simulink model "gm_model"  (R2022a)
settings: Solver=FixedStepAuto  StartTime=0.0  StopTime=1e2  RelTol=1e-3
settings Model: Creator=mrem  LastModifiedBy=mrem
settings OptimizationCC: BlockReduction=off  ConditionallyExecuteInputs=off
settings DebuggingCC: InheritedTsInSrcMsg=none

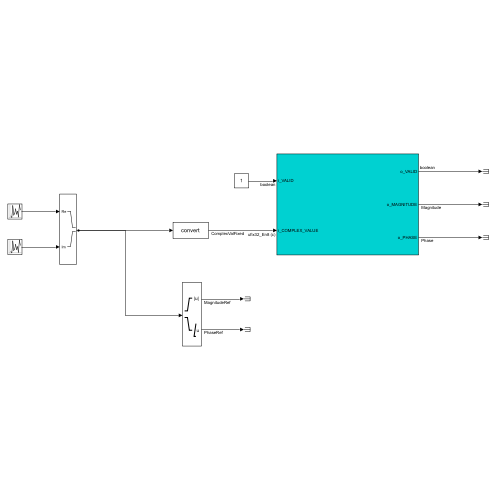
[thumbnail: Simulink's stored preview of the top-level diagram]
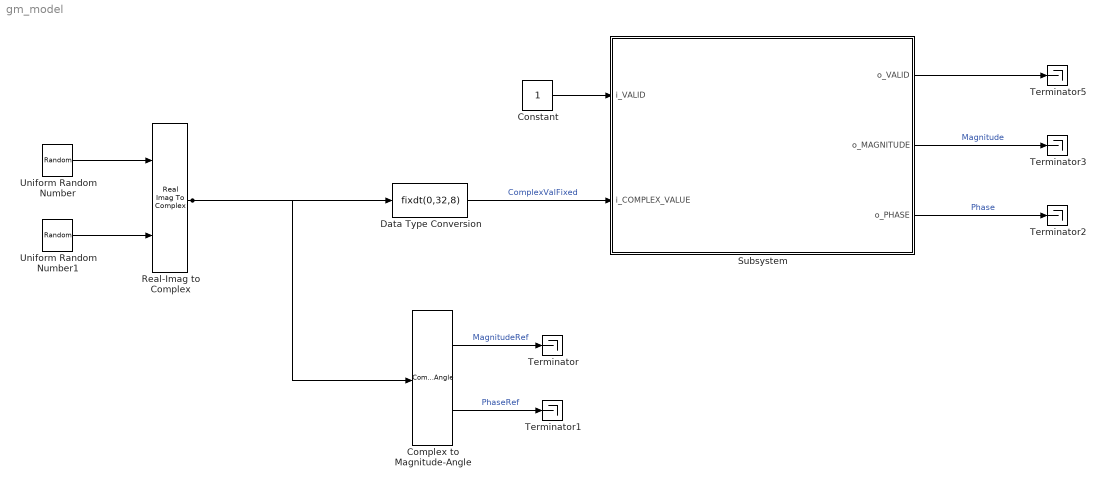
== system gm_model ==
  Complex to Magnitude-Angle : ComplexToMagnitudeAngle
  Constant : Constant  OutDataTypeStr=boolean  SampleTime=-1
  Data Type Conversion : DataTypeConversion  OutDataTypeStr=fixdt(0,32,8)  RndMeth=Round  SaturateOnIntegerOverflow=off
  Real-Imag to Complex : RealImagToComplex
  Subsystem : Subsystem
  Terminator{,1..3,5} (5 alike) : Terminator
  Uniform Random Number : UniformRandomNumber  Minimum=0  Maximum=16777215.9909375  Seed=24  SampleTime=1
  Uniform Random Number1 : UniformRandomNumber  Minimum=0  Maximum=16777215.9909375  Seed=25  SampleTime=1
  wires:
  Data Type Conversion/1 -> Subsystem/2(i_COMPLEX_VALUE)  "ComplexValFixed"
  Subsystem/1(o_VALID) -> Terminator5/1
  Subsystem/3(o_PHASE) -> Terminator2/1  "Phase"
  Subsystem/2(o_MAGNITUDE) -> Terminator3/1  "Magnitude"
  Complex to Magnitude-Angle/2 -> Terminator1/1  "PhaseRef"
  Complex to Magnitude-Angle/1 -> Terminator/1  "MagnitudeRef"
  Real-Imag to Complex/1 -> Data Type Conversion/1, Complex to Magnitude-Angle/1
  Uniform Random Number/1 -> Real-Imag to Complex/1
  Uniform Random Number1/1 -> Real-Imag to Complex/2
  Constant/1 -> Subsystem/1(i_VALID)

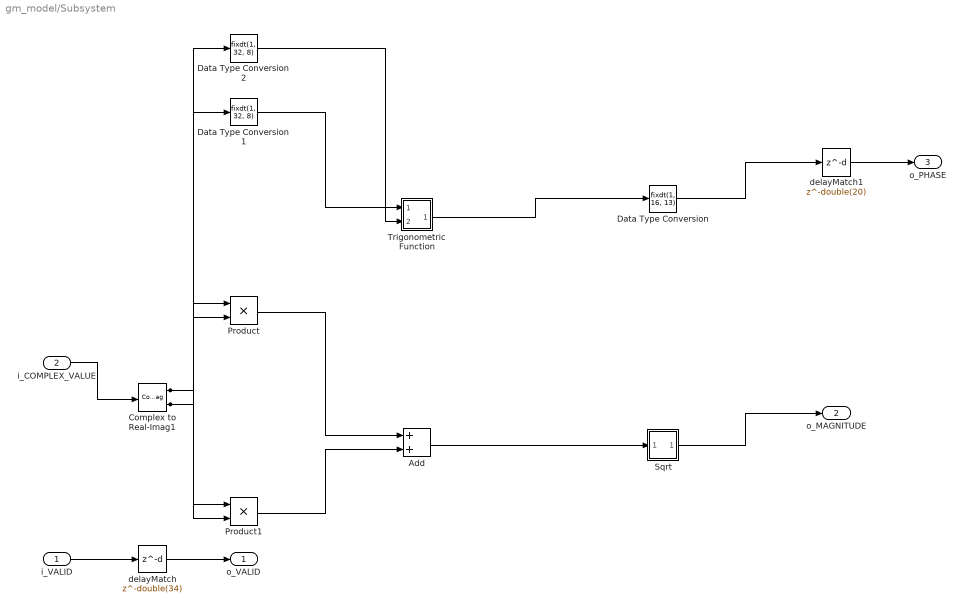
== system gm_model/Subsystem ==
  i_VALID : Inport  OutDataTypeStr=boolean  PortDimensions=1  SampleTime=1
  i_COMPLEX_VALUE : Inport  Port=2  OutDataTypeStr=fixdt(0, 32, 8)  PortDimensions=1  SampleTime=1  LockScale=on
      settings: SignalType=complex
  Add : Sum  AccumDataTypeStr=fixdt(0, 64, 16)  OutDataTypeStr=fixdt(0, 64, 16)  SampleTime=1
  Complex to Real-Imag1 : ComplexToRealImag  SampleTime=1
  Data Type Conversion : DataTypeConversion  OutDataTypeStr=fixdt(1, 16, 13)  SampleTime=1  SaturateOnIntegerOverflow=off  RndMeth=Floor
  Data Type Conversion1 : DataTypeConversion  OutDataTypeStr=fixdt(1, 32, 8)  SampleTime=1  SaturateOnIntegerOverflow=off  RndMeth=Floor
  Data Type Conversion2 : DataTypeConversion  OutDataTypeStr=fixdt(1, 32, 8)  SampleTime=1  SaturateOnIntegerOverflow=off  RndMeth=Floor
  Product : Product  Inputs=**  OutDataTypeStr=fixdt(0, 64, 16)  SampleTime=1
  Product1 : Product  Inputs=**  OutDataTypeStr=fixdt(0, 64, 16)  SampleTime=1
  Sqrt : Subsystem
  Trigonometric Function : Subsystem
  delayMatch : Delay  DelayLength=double(34)  InitialCondition=0  SampleTime=1
  delayMatch1 : Delay  DelayLength=double(20)  InitialCondition=0  SampleTime=1
  o_VALID : Outport  OutDataTypeStr=boolean  SampleTime=1
  o_MAGNITUDE : Outport  Port=2  SampleTime=1
  o_PHASE : Outport  Port=3  SampleTime=1
  wires:
  delayMatch/1 -> o_VALID/1
  i_COMPLEX_VALUE/1 -> Complex to Real-Imag1/1
  Add/1 -> Sqrt/1(In1)
  Complex to Real-Imag1/1 -> Product/2, Product/1, Data Type Conversion2/1
  Complex to Real-Imag1/2 -> Product1/2, Product1/1, Data Type Conversion1/1
  delayMatch1/1 -> o_PHASE/1
  Data Type Conversion1/1 -> Trigonometric Function/1(In1)
  Data Type Conversion2/1 -> Trigonometric Function/2(In2)
  Product/1 -> Add/1
  Product1/1 -> Add/2
  Sqrt/1(Out1) -> o_MAGNITUDE/1
  Trigonometric Function/1(Out1) -> Data Type Conversion/1
  i_VALID/1 -> delayMatch/1
  Data Type Conversion/1 -> delayMatch1/1

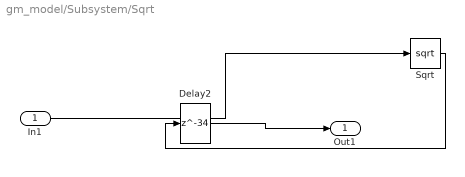
== system gm_model/Subsystem/Sqrt ==
  In1 : Inport
  Delay2 : Delay  DelayLength=34
  Sqrt : Sqrt  OutDataTypeStr=fixdt(0,33,8)
  Out1 : Outport
  wires:
  In1/1 -> Sqrt/1
  Sqrt/1 -> Delay2/1
  Delay2/1 -> Out1/1

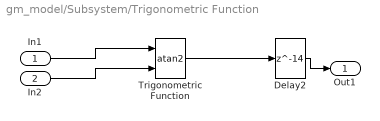
== system gm_model/Subsystem/Trigonometric Function ==
  In1 : Inport
  In2 : Inport  Port=2
  Delay2 : Delay  DelayLength=14
  Trigonometric Function : Trigonometry  Operator=atan2  ApproximationMethod=CORDIC
  Out1 : Outport
  wires:
  In1/1 -> Trigonometric Function/1
  In2/1 -> Trigonometric Function/2
  Trigonometric Function/1 -> Delay2/1
  Delay2/1 -> Out1/1
